simulink model "SkywalkerX8_Control_Digital"  (R2018a)
settings: Solver=FixedStepAuto  StartTime=0.0  StopTime=120  FixedStep=0.001  RelTol=1e-3
undefined symbols (not defined in the file): DiscIntNeverNeededParam, sigbuilder_block, SkywalkerX8
libraries: simulink_extras x9, simulink x3
(part 1 of 2)
settings Model: Creator=David  LastModifiedBy=David
settings OptimizationCC: DefaultParameterBehavior=Inlined  EnhancedBackFolding=on  PassReuseOutputArgsThreshold=0  OptimizeBlockOrder=speed  DifferentSizesBufferReuse=on  OptimizationCustomize=off
settings DebuggingCC: ParameterTunabilityLossMsg=error
settings SFSimCC: MATLABDynamicMemAlloc=off
settings RTWCC: GenCodeOnly=on  Description=Generic Real-Time Target  GenerateReport=on  LaunchReport=on
settings CodeAppCC: ForceParamTrailComments=on  OperatorAnnotations=on

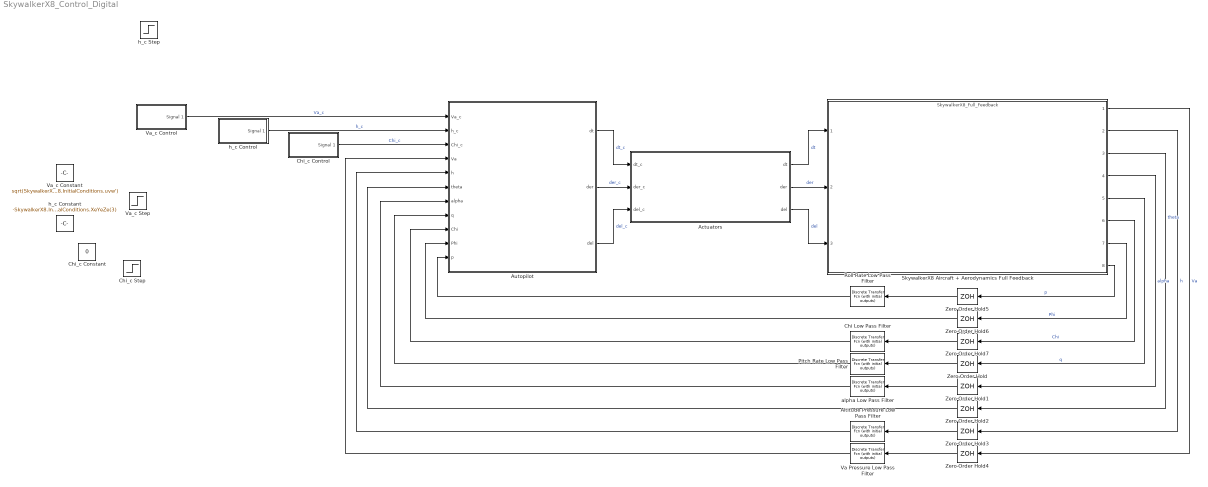
== system SkywalkerX8_Control_Digital ==
  Actuators : Subsystem
      mask Display:
      | image('actuators.jpg', 'center')
      | 
      | color('white')
      | 
      | port_label('input', 1, 'd_{t_c} (Unitless)', 'texmode', 'on')
      | port_label('input', 2, 'd_{{er}_c} (rad)', 'texmode', 'on')
      | port_label('input', 3, 'd_{{el}_c} (rad)', 'texmode', 'on')
      | 
      | port_label('output', 1, 'd_t (Unitless)', 'texmode', 'on')
      | port_label('output', 2, 'd_{er} (rad)', 'texmode', 'on')
      | port_label('output', 3, 'd_{el} (rad)', 'texmode', 'on')
  Altitude Pressure Low Pass Filter : simulink_extras/Additional Discrete/Discrete Transfer Fcn (with initial outputs)  N=cell2mat(SkywalkerX8.Sensors.Filters.AltitudePressure.FilterTFDigital.Numerator)  D=cell2mat(SkywalkerX8.Sensors.Filters.AltitudePressure.FilterTFDigital.Denominator)  U0=-SkywalkerX8.InitialConditions.XeYeZe(3)  Y0=-SkywalkerX8.InitialConditions.XeYeZe(3)  TS=SkywalkerX8.Sensors.Filters.AltitudePressure.FilterSampleTime
      settings: SourceProductName=Simulink  SourceProductBaseCode=SL
  Autopilot : Subsystem
      mask Display:
      | image('autopilot.png', 'center')
      | 
      | port_label('output', 1, '\delta_t (Unitless)', 'texmode', 'on')
      | port_label('output', 2, '\delta_e_r (rad)', 'texmode', 'on')
      | port_label('output', 3, '\delta_e_l (rad)', 'texmode', 'on')
      | 
      | port_label('input', 1, 'V_{a_c} (m/s)', 'texmode', 'on')
      | port_label('input', 2, 'h_c (m)', 'texmode', 'on')
      | port_label('input', 3, '\chi_c (rad)', 'texmode', 'on')
      | port_label('input', 4, 'V_a (m/s)', 'texmode', 'on')
      | port_label('input', 5, 'Altitude (m)', 'texmode', 'on')
      | port_label('input', 6, '\theta (rad)', 'texmode', 'on')
      | port_label('input', 7, '\alpha (rad)', 'texmode', 'on')
      | port_label('input', 8, 'q (rad/s)', 'texmode', 'on')
      | port_label('input', 9, '\chi (rad)', 'texmode', 'on')
      | port_label('input', 10, '\phi (rad)', 'texmode', 'on')
      | port_label('input', 11, 'p (rad/s)', 'texmode', 'on')
  Chi Low Pass Filter : simulink_extras/Additional Discrete/Discrete Transfer Fcn (with initial outputs)  N=cell2mat(SkywalkerX8.Sensors.EKF.GPSSmoothing.Filters.ChiFilter.TFDigital.Numerator)  D=cell2mat(SkywalkerX8.Sensors.EKF.GPSSmoothing.Filters.ChiFilter.TFDigital.Denominator)  U0=SkywalkerX8.Sensors.EKF.GPSSmoothing.Filters.ChiFilter.InitialCondition  Y0=SkywalkerX8.Sensors.EKF.GPSSmoothing.Filters.ChiFilter.InitialCondition  TS=SkywalkerX8.Sensors.EKF.GPSSmoothing.Filters.ChiFilter.SampleTime
      settings: SourceProductName=Simulink  SourceProductBaseCode=SL
  Chi_c Constant : Constant  Value=0
  Chi_c Control : Subsystem  Tag=STV Subsys  LoadFcn=sigbuilder_block('load');  StartFcn=sigbuilder_block('start');  StopFcn=sigbuilder_block('stop');  ClipboardFcn=sigbuilder_block('clipboard');  mask(Sigbuilder block){tuvar=[0:10]}
      mask help: Simulink:masks:SigbuilderBlock_MD
      mask init:
      | if ~strcmp(get_param(bdroot(gcbh),'SimulationStatus'),'stopped') tuvar = sigbuilder_block('maskInit'); end
      settings: CopyFcn=sigbuilder_block('copy');  DeleteFcn=sigbuilder_block('delete');  ModelCloseFcn=sigbuilder_block('modelClose');  PreSaveFcn=sigbuilder_block('preSave');  PauseFcn=sigbuilder_block('pause');  ContinueFcn=sigbuilder_block('continue');  NameChangeFcn=sigbuilder_block('namechange');  OpenFcn=sigbuilder_block('open',[437.6 199.2 550.4 400 ]);  CloseFcn=sigbuilder_block('close');
      mask Display: plot(0, 0, 100, 100,[2, 2, 32, 32, 2], [68, 8, 8, 68, 68],[32, 2], [38, 38], [32, 19, 2],[53, 60, 44], [32, 17, 17, 2],[16, 16, 31, 31]);txt = getActiveGroup(gcbh);text(2, 100, txt,'verticalAlignment', 'top');
  Chi_c Step : Step  After=deg2rad(90)  SampleTime=0
  Pitch Rate Low Pass Filter : simulink_extras/Additional Discrete/Discrete Transfer Fcn (with initial outputs)  N=cell2mat(SkywalkerX8.Sensors.Filters.AngularRates.Pitch.FilterTFDigital.Numerator)  D=cell2mat(SkywalkerX8.Sensors.Filters.AngularRates.Pitch.FilterTFDigital.Denominator)  U0=SkywalkerX8.Sensors.Filters.AngularRates.Pitch.InitialCondition  Y0=SkywalkerX8.Sensors.Filters.AngularRates.Pitch.InitialCondition  TS=SkywalkerX8.Sensors.Filters.AngularRates.Pitch.FilterSampleTime
      settings: SourceProductName=Simulink  SourceProductBaseCode=SL
  Roll Rate Low Pass Filter : simulink_extras/Additional Discrete/Discrete Transfer Fcn (with initial outputs)  N=cell2mat(SkywalkerX8.Sensors.Filters.AngularRates.Roll.FilterTFDigital.Numerator)  D=cell2mat(SkywalkerX8.Sensors.Filters.AngularRates.Roll.FilterTFDigital.Denominator)  U0=SkywalkerX8.Sensors.Filters.AngularRates.Roll.InitialCondition  Y0=SkywalkerX8.Sensors.Filters.AngularRates.Roll.InitialCondition  TS=SkywalkerX8.Sensors.Filters.AngularRates.Roll.FilterSampleTime
      settings: SourceProductName=Simulink  SourceProductBaseCode=SL
  SkywalkerX8 Aircraft + Aerodynamics Full Feedback : ModelReference  ModelNameDialog=SkywalkerX8_Full_Feedback  ModelReferenceVersion=1.30
      mask Display:
      | image('x8SkySunset.png', 'center')
      | 
      | port_label('input', 1, '\delta_t (Unitless)', 'texmode', 'on')
      | port_label('input', 2, '\delta_e_r (rad)', 'texmode', 'on')
      | port_label('input', 3, '\delta_e_l (rad)', 'texmode', 'on')
      | 
      | port_label('output', 1, 'V_a (m/s)', 'texmode', 'on')
      | port_label('output', 2, 'Altitude (m)', 'texmode', 'on')
      | port_label('output', 3, '\theta (rad)', 'texmode', 'on')
      | port_label('output', 4, '\alpha (rad)', 'texmode', 'on')
      | port_label('output', 5, 'q (rad/s)', 'texmode', 'on')
      | port_label('output', 6, '\chi (rad)', 'texmode', 'on')
      | port_label('output', 7, '\phi (rad)', 'texmode', 'on')
      | port_label('output', 8, 'p (rad/s)', 'texmode', 'on')
  Va Pressure Low Pass Filter : simulink_extras/Additional Discrete/Discrete Transfer Fcn (with initial outputs)  N=cell2mat(SkywalkerX8.Sensors.Filters.AirspeedPressure.FilterTFDigital.Numerator)  D=cell2mat(SkywalkerX8.Sensors.Filters.AirspeedPressure.FilterTFDigital.Denominator)  U0=sqrt(SkywalkerX8.InitialConditions.uvw*SkywalkerX8.InitialConditions.uvw')  Y0=sqrt(SkywalkerX8.InitialConditions.uvw*SkywalkerX8.InitialConditions.uvw')  TS=SkywalkerX8.Sensors.Filters.AirspeedPressure.FilterSampleTime
      settings: SourceProductName=Simulink  SourceProductBaseCode=SL
  Va_c Constant : Constant  Value=sqrt(SkywalkerX8.InitialConditions.uvw*SkywalkerX8.InitialConditions.uvw')
  Va_c Control : Subsystem  Tag=STV Subsys  LoadFcn=sigbuilder_block('load');  StartFcn=sigbuilder_block('start');  StopFcn=sigbuilder_block('stop');  ClipboardFcn=sigbuilder_block('clipboard');  mask(Sigbuilder block){tuvar=[0:10]}
      mask help: Simulink:masks:SigbuilderBlock_MD
      mask init:
      | if ~strcmp(get_param(bdroot(gcbh),'SimulationStatus'),'stopped') tuvar = sigbuilder_block('maskInit'); end
      settings: CopyFcn=sigbuilder_block('copy');  DeleteFcn=sigbuilder_block('delete');  ModelCloseFcn=sigbuilder_block('modelClose');  PreSaveFcn=sigbuilder_block('preSave');  PauseFcn=sigbuilder_block('pause');  ContinueFcn=sigbuilder_block('continue');  NameChangeFcn=sigbuilder_block('namechange');  OpenFcn=sigbuilder_block('open',[437.6 199.2 550.4 400 ]);  CloseFcn=sigbuilder_block('close');
      mask Display: plot(0, 0, 100, 100,[2, 2, 32, 32, 2], [68, 8, 8, 68, 68],[32, 2], [38, 38], [32, 19, 2],[53, 60, 44], [32, 17, 17, 2],[16, 16, 31, 31]);txt = getActiveGroup(gcbh);text(2, 100, txt,'verticalAlignment', 'top');
  Va_c Step : Step  Before=sqrt(SkywalkerX8.InitialConditions.uvw*SkywalkerX8.InitialConditions.uvw')  After=sqrt(SkywalkerX8.InitialConditions.uvw*SkywalkerX8.InitialConditions.uvw')  SampleTime=0
  Zero-Order Hold : ZeroOrderHold  SampleTime=SkywalkerX8.Sensors.IMU.Gyroscope.SampleTime
  Zero-Order Hold1 : ZeroOrderHold  SampleTime=SkywalkerX8.Sensors.AoA.SampleTime
  Zero-Order Hold2 : ZeroOrderHold  SampleTime=SkywalkerX8.Sensors.EKF.GPSSmoothing.StateTransitionSampleTime
  Zero-Order Hold3 : ZeroOrderHold  SampleTime=SkywalkerX8.Sensors.AltitudePressure.SampleTime
  Zero-Order Hold4 : ZeroOrderHold  SampleTime=SkywalkerX8.Sensors.AirspeedPressure.SampleTime
  Zero-Order Hold5 : ZeroOrderHold  SampleTime=SkywalkerX8.Sensors.IMU.Gyroscope.SampleTime
  Zero-Order Hold6 : ZeroOrderHold  SampleTime=SkywalkerX8.Sensors.EKF.Attitude.StateTransitionSampleTime
  Zero-Order Hold7 : ZeroOrderHold  SampleTime=SkywalkerX8.Sensors.EKF.GPSSmoothing.StateTransitionSampleTime
  alpha Low Pass Filter : simulink_extras/Additional Discrete/Discrete Transfer Fcn (with initial outputs)  N=cell2mat(SkywalkerX8.Sensors.Filters.AoA.FilterTFDigital.Numerator)  D=cell2mat(SkywalkerX8.Sensors.Filters.AoA.FilterTFDigital.Denominator)  U0=SkywalkerX8.Sensors.Filters.AoA.InitialCondition  Y0=SkywalkerX8.Sensors.Filters.AoA.InitialCondition  TS=SkywalkerX8.Sensors.Filters.AoA.FilterSampleTime
      settings: SourceProductName=Simulink  SourceProductBaseCode=SL
  h_c Constant : Constant  Value=-SkywalkerX8.InitialConditions.XeYeZe(3)
  h_c Control : Subsystem  Tag=STV Subsys  LoadFcn=sigbuilder_block('load');  StartFcn=sigbuilder_block('start');  StopFcn=sigbuilder_block('stop');  ClipboardFcn=sigbuilder_block('clipboard');  mask(Sigbuilder block){tuvar=[0:10]}
      mask help: Simulink:masks:SigbuilderBlock_MD
      mask init:
      | if ~strcmp(get_param(bdroot(gcbh),'SimulationStatus'),'stopped') tuvar = sigbuilder_block('maskInit'); end
      settings: CopyFcn=sigbuilder_block('copy');  DeleteFcn=sigbuilder_block('delete');  ModelCloseFcn=sigbuilder_block('modelClose');  PreSaveFcn=sigbuilder_block('preSave');  PauseFcn=sigbuilder_block('pause');  ContinueFcn=sigbuilder_block('continue');  NameChangeFcn=sigbuilder_block('namechange');  OpenFcn=sigbuilder_block('open',[6 30 1428 771.75 ]);  CloseFcn=sigbuilder_block('close');
      mask Display: plot(0, 0, 100, 100,[2, 2, 32, 32, 2], [68, 8, 8, 68, 68],[32, 2], [38, 38], [32, 19, 2],[53, 60, 44], [32, 17, 17, 2],[16, 16, 31, 31]);txt = getActiveGroup(gcbh);text(2, 100, txt,'verticalAlignment', 'top');
  h_c Step : Step  Time=0.1  Before=-SkywalkerX8.InitialConditions.XeYeZe(3)  After=100  SampleTime=0
  wires:
  SkywalkerX8 Aircraft + Aerodynamics Full Feedback/6 -> Zero-Order Hold7/1  "Chi"
  SkywalkerX8 Aircraft + Aerodynamics Full Feedback/5 -> Zero-Order Hold/1  "q"
  SkywalkerX8 Aircraft + Aerodynamics Full Feedback/4 -> Zero-Order Hold1/1  "alpha"
  SkywalkerX8 Aircraft + Aerodynamics Full Feedback/3 -> Zero-Order Hold2/1  "theta"
  SkywalkerX8 Aircraft + Aerodynamics Full Feedback/2 -> Zero-Order Hold3/1  "h"
  SkywalkerX8 Aircraft + Aerodynamics Full Feedback/1 -> Zero-Order Hold4/1  "Va"
  Zero-Order Hold5/1 -> Roll Rate Low Pass Filter/1
  Zero-Order Hold6/1 -> Autopilot/10(Phi)
  Zero-Order Hold7/1 -> Chi Low Pass Filter/1
  Zero-Order Hold/1 -> Pitch Rate Low Pass Filter/1
  Zero-Order Hold1/1 -> alpha Low Pass Filter/1
  Zero-Order Hold2/1 -> Autopilot/6(theta)
  Zero-Order Hold3/1 -> Altitude Pressure Low Pass Filter/1
  Zero-Order Hold4/1 -> Va Pressure Low Pass Filter/1
  h_c Control/1(Signal 1) -> Autopilot/2(h_c)  "h_c"
  Chi_c Control/1(Signal 1) -> Autopilot/3(Chi_c)  "Chi_c"
  Va_c Control/1(Signal 1) -> Autopilot/1(Va_c)  "Va_c"
  SkywalkerX8 Aircraft + Aerodynamics Full Feedback/8 -> Zero-Order Hold5/1  "p"
  SkywalkerX8 Aircraft + Aerodynamics Full Feedback/7 -> Zero-Order Hold6/1  "Phi"
  Autopilot/1(dt) -> Actuators/1(dt_c)  "dt_c"
  Actuators/1(dt) -> SkywalkerX8 Aircraft + Aerodynamics Full Feedback/1  "dt"
  Autopilot/2(der) -> Actuators/2(der_c)  "der_c"
  Actuators/2(der) -> SkywalkerX8 Aircraft + Aerodynamics Full Feedback/2  "der"
  Autopilot/3(del) -> Actuators/3(del_c)  "del_c"
  Actuators/3(del) -> SkywalkerX8 Aircraft + Aerodynamics Full Feedback/3  "del"
  Roll Rate Low Pass Filter/1 -> Autopilot/11(p)
  alpha Low Pass Filter/1 -> Autopilot/7(alpha)
  Altitude Pressure Low Pass Filter/1 -> Autopilot/5(h)
  Va Pressure Low Pass Filter/1 -> Autopilot/4(Va)
  Pitch Rate Low Pass Filter/1 -> Autopilot/8(q)
  Chi Low Pass Filter/1 -> Autopilot/9(Chi)

== system SkywalkerX8_Control_Digital/Actuators ==
  dt_c : Inport
  der_c : Inport  Port=2
  del_c : Inport  Port=3
  Left Servo-Motor : Subsystem
      mask Display: image('servo.jpg', 'center')
  Motor Model : simulink_extras/Additional Linear/State-Space (with initial outputs)  A=SkywalkerX8.Actuators.Motor.SS.A  B=SkywalkerX8.Actuators.Motor.SS.B  C=SkywalkerX8.Actuators.Motor.SS.C  D=SkywalkerX8.Actuators.Motor.SS.D  U0=SkywalkerX8.InitialConditions.dt  Y0=SkywalkerX8.InitialConditions.dt  mask(State-Space with Initial Outputs){}
      settings: SourceProductName=Simulink  SourceProductBaseCode=SL
      mask Display: image('motor.jpg', 'center')
  Right Servo-Motor : Subsystem
      mask Display: image('servo.jpg', 'center')
  dt : Outport
  der : Outport  Port=2
  del : Outport  Port=3
  wires:
  del_c/1 -> Left Servo-Motor/1(del_c)
  Motor Model/1 -> dt/1
  Left Servo-Motor/1(del) -> del/1
  der_c/1 -> Right Servo-Motor/1(der_c)
  dt_c/1 -> Motor Model/1
  Right Servo-Motor/1(der) -> der/1

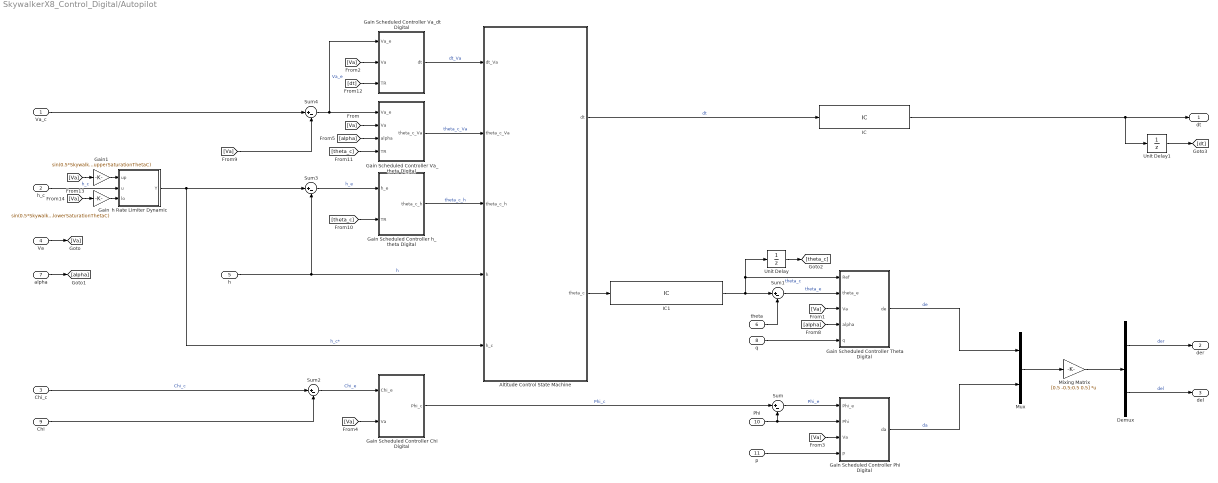
== system SkywalkerX8_Control_Digital/Autopilot ==
  Va_c : Inport
  h_c : Inport  Port=2
  Chi_c : Inport  Port=3
  Va : Inport  Port=4
  h : Inport  Port=5
  theta : Inport  Port=6
  alpha : Inport  Port=7
  q : Inport  Port=8
  Chi : Inport  Port=9
  Phi : Inport  Port=10
  p : Inport  Port=11
  Altitude Control State Machine : Stateflow chart  TreatAsAtomicUnit=on  mask{h_hold=SkywalkerX8.Control.Longitudinal.AltStateMachine.hHold, h_takeoff=SkywalkerX8.Control.Longitudinal.AltStateMachine.hTakeOff, theta_c_takeoff=SkywalkerX8.Control.Longitudinal.AltStateMachine.thetaTakeOff, hyst_frac=SkywalkerX8.Control.Longitudinal.AltStateMachine.HysteresisFraction, PreFlightBypass=SkywalkerX8.Control.Longitudinal.AltStateMachine.PreFlightBypass}
      mask prompts: h_hold "Altitude hold zone (+- band around the commanded altitude where theta will control altitude) (m)"; h_takeoff "Takeoff altitude (altitude after which we move away from constant pitch angle command) (m)"; theta_c_takeoff "Takeoff pitch angle (constant pitch angle at which to climb at at takeoff) (rad)"; hyst_frac "Hysteresis Fraction (Unitless)"; PreFlightBypass "Preflight Bypass (Unitless)"
  Demux : Demux  Outputs=2
  Gain : Gain  Gain=sin(0.5*SkywalkerX8.Control.Longitudinal.altController.lowerSaturationThetaC)
  Gain Scheduled Controller Chi Digital : Subsystem
  Gain Scheduled Controller Phi Digital : Subsystem
  Gain Scheduled Controller Theta Digital : Subsystem
  Gain Scheduled Controller Va_dt Digital : Subsystem
  Gain Scheduled Controller Va_theta Digital : Subsystem
  Gain Scheduled Controller h_theta Digital : Subsystem
  Gain1 : Gain  Gain=sin(0.5*SkywalkerX8.Control.Longitudinal.altController.upperSaturationThetaC)
  IC : InitialCondition  Value=SkywalkerX8.InitialConditions.dt
  IC1 : InitialCondition  Value=SkywalkerX8.InitialConditions.PhiThetaPsi(2)
  Mixing Matrix : Gain  Gain=[0.5 -0.5;0.5 0.5]  Multiplication=Matrix(K*u)
  Mux : Mux  Inputs=2
  Sum{,1..4} (5 alike) : Sum  Inputs=|+-
  Unit Delay : UnitDelay  InitialCondition=SkywalkerX8.InitialConditions.PhiThetaPsi(2)  SampleTime=SkywalkerX8.Control.Longitudinal.thetaController.Digital.SampleTime
  Unit Delay1 : UnitDelay  InitialCondition=SkywalkerX8.InitialConditions.dt  SampleTime=SkywalkerX8.Control.Longitudinal.VaDtController.Digital.SampleTime
  h Rate Limiter Dynamic : Subsystem  mask{initOutput=-SkywalkerX8.InitialConditions.XeYeZe(3)}
      mask prompts: initOutput "Initial output of dynamic rate limiter"
      mask DialogControl DescGroupVar Prompt: Rate Limiter Dynamic
      mask DialogControl DescTextVar Prompt: Limit rising and falling rates of the signals at the second input by using the first input (upper limit) and the third input (lower limit).
      mask Display:
      | image('rateLimit.png')
      | 
      | port_label('input', 1, 'up')
      | port_label('input', 2, 'u')
      | port_label('input', 3, 'lo')
      | 
      | port_label('output', 1, 'Y')
  dt : Outport
  der : Outport  Port=2
  del : Outport  Port=3
  wires:
  [Va] -> Sum4/2
  Sum4/1 -> Gain Scheduled Controller Va_theta Digital/1(Va_e), Gain Scheduled Controller Va_dt Digital/1(Va_e)  "Va_e"
  Demux/1 -> der/1  "der"
  Gain Scheduled Controller Chi Digital/1(Phi_c) -> Sum/1  "Phi_c"
  h/1 -> Altitude Control State Machine/4(h), Sum3/2  "h"
  h Rate Limiter Dynamic/1(Y) -> Altitude Control State Machine/5(h_c), Sum3/1  "h_c*"
  Sum3/1 -> Gain Scheduled Controller h_theta Digital/1(h_e)  "h_e"
  Sum2/1 -> Gain Scheduled Controller Chi Digital/1(Chi_e)  "Chi_e"
  Phi/1 -> Gain Scheduled Controller Phi Digital/2(Phi), Sum/2
  Sum/1 -> Gain Scheduled Controller Phi Digital/1(Phi_e)  "Phi_e"
  Gain Scheduled Controller Phi Digital/1(da) -> Mux/2  "da"
  [Va] -> Gain Scheduled Controller Phi Digital/3(Va)
  [Va] -> Gain Scheduled Controller Theta Digital/3(Va)
  [alpha] -> Gain Scheduled Controller Va_theta Digital/3(alpha)
  [Va] -> Gain Scheduled Controller Chi Digital/2(Va)
  Sum1/1 -> Gain Scheduled Controller Theta Digital/2(theta_e)  "theta_e"
  [Va] -> Gain Scheduled Controller Va_dt Digital/2(Va)
  Demux/2 -> del/1  "del"
  alpha/1 -> [alpha]
  [Va] -> Gain Scheduled Controller Va_theta Digital/2(Va)
  Chi/1 -> Sum2/2
  Gain Scheduled Controller Theta Digital/1(de) -> Mux/1  "de"
  p/1 -> Gain Scheduled Controller Phi Digital/4(p)
  Va/1 -> [Va]
  theta/1 -> Sum1/2
  Mux/1 -> Mixing Matrix/1
  Mixing Matrix/1 -> Demux/1
  Altitude Control State Machine/1(dt) -> IC/1  "dt"
  Gain Scheduled Controller Va_theta Digital/1(theta_c_Va) -> Altitude Control State Machine/2(theta_c_Va)  "theta_c_Va"
  [theta_c] -> Gain Scheduled Controller Va_theta Digital/4(TR)
  [dt] -> Gain Scheduled Controller Va_dt Digital/3(TR)
  IC/1 -> Unit Delay1/1, dt/1
  [theta_c] -> Gain Scheduled Controller h_theta Digital/2(TR)
  IC1/1 -> Gain Scheduled Controller Theta Digital/1(Ref), Unit Delay/1, Sum1/1  "theta_c"
  [alpha] -> Gain Scheduled Controller Theta Digital/4(alpha)
  q/1 -> Gain Scheduled Controller Theta Digital/5(q)
  Gain Scheduled Controller h_theta Digital/1(theta_c_h) -> Altitude Control State Machine/3(theta_c_h)  "theta_c_h"
  Altitude Control State Machine/2(theta_c) -> IC1/1
  Gain Scheduled Controller Va_dt Digital/1(dt) -> Altitude Control State Machine/1(dt_Va)  "dt_Va"
  h_c/1 -> h Rate Limiter Dynamic/2(u)  "h_c"
  [Va] -> Gain1/1
  Gain/1 -> h Rate Limiter Dynamic/3(lo)
  [Va] -> Gain/1
  Gain1/1 -> h Rate Limiter Dynamic/1(up)
  Chi_c/1 -> Sum2/1  "Chi_c"
  Va_c/1 -> Sum4/1
  Unit Delay/1 -> [theta_c]
  Unit Delay1/1 -> [dt]

== system SkywalkerX8_Control_Digital/Chi_c Control ==
  Demux : Demux  Tag=STV Demux  Outputs=1
  FromWs : FromWorkspace  Tag=STV FromWs  VariableName=tuvar  SampleTime=0
      SigBuilderData=|
      | common.afterFinalStr = 'Extrapolate'
      | common.sampleTime = 0
      | dataSet.timeRange = [0 120]
      | dataSet.name = 'Group 1'
      | sbobj.Groups.Name = 'Group 1'
      | sbobj.Groups.Signals.Name = 'Signal 1'
      | sbobj.Groups.Signals.XData = [0 10 10 35 35 55 55 90 90 120]
      | sbobj.Groups.Signals.YData = [0 0 1.5708 1.5708 0 0 1.5708 1.5708 0 0]
      | sbobj.Groups.TimeRange = [0 120]
  Signal 1 : Outport  Tag=STV Outport
  wires:
  Demux/1 -> Signal 1/1
  FromWs/1 -> Demux/1

== system SkywalkerX8_Control_Digital/Va_c Control ==
  Demux : Demux  Tag=STV Demux  Outputs=1
  FromWs : FromWorkspace  Tag=STV FromWs  VariableName=tuvar  SampleTime=0
      SigBuilderData=|
      | common.afterFinalStr = 'Extrapolate'
      | common.sampleTime = 0
      | dataSet.timeRange = [0 120]
      | dataSet.name = 'Group 1'
      | sbobj.Groups.Name = 'Group 1'
      | sbobj.Groups.Signals.Name = 'Signal 1'
      | sbobj.Groups.Signals.XData = [0 10 10 30 30 50 50 70 70 120]
      | sbobj.Groups.Signals.YData = [17.3072 17.3 20 20 17.3072 17.3072 15 15 17.3072 17.3072]
      | sbobj.Groups.TimeRange = [0 120]
  Signal 1 : Outport  Tag=STV Outport
  wires:
  Demux/1 -> Signal 1/1
  FromWs/1 -> Demux/1

== system SkywalkerX8_Control_Digital/h_c Control ==
  Demux : Demux  Tag=STV Demux  Outputs=1
  FromWs : FromWorkspace  Tag=STV FromWs  VariableName=tuvar  SampleTime=0
      SigBuilderData=|
      | common.afterFinalStr = 'Extrapolate'
      | common.sampleTime = 0
      | dataSet.timeRange = [0 120]
      | dataSet.name = 'Group 1'
      | sbobj.Groups.Name = 'Group 1'
      | sbobj.Groups.Signals.Name = 'Signal 1'
      | sbobj.Groups.Signals.XData = [0 1 1 20 20 40 40 60 80 80 100 100 120]
      | sbobj.Groups.Signals.YData = [50 50 60 60 75 75 100 100 80 60 60 100 100]
      | sbobj.Groups.TimeRange = [0 120]
  Signal 1 : Outport  Tag=STV Outport
  wires:
  Demux/1 -> Signal 1/1
  FromWs/1 -> Demux/1

== system SkywalkerX8_Control_Digital/Actuators/Left Servo-Motor ==
  del_c : Inport
  Abs : Abs
  Compare To Constant : simulink/Logic and Bit Operations/Compare To Constant  relop=>  const=SkywalkerX8.Actuators.Servos.RateLimit  OutDataTypeStr=boolean
  Derivative : Derivative
  Rate Limiter : RateLimiter  Commented=through  RisingSlewLimit=SkywalkerX8.Actuators.Servos.RateLimit  FallingSlewLimit=-SkywalkerX8.Actuators.Servos.RateLimit  SampleTimeMode=inherited  InitialCondition=SkywalkerX8.InitialConditions.de*0.5 + SkywalkerX8.InitialConditions.da*0.5
  Saturation : Saturate  UpperLimit=SkywalkerX8.Actuators.Servos.UpperSaturation  LowerLimit=SkywalkerX8.Actuators.Servos.LowerSaturation
  Second Order Servo-Motor Model : simulink_extras/Additional Linear/State-Space (with initial outputs)  A=SkywalkerX8.Actuators.Servos.SS.A  B=SkywalkerX8.Actuators.Servos.SS.B  C=SkywalkerX8.Actuators.Servos.SS.C  D=SkywalkerX8.Actuators.Servos.SS.D  U0=(SkywalkerX8.InitialConditions.de*0.5 + SkywalkerX8.InitialConditions.da*0.5)  Y0=(SkywalkerX8.InitialConditions.de*0.5 + SkywalkerX8.InitialConditions.da*0.5)
      settings: SourceProductName=Simulink  SourceProductBaseCode=SL
  Terminator : Terminator
  del : Outport
  wires:
  Rate Limiter/1 -> Saturation/1
  del_c/1 -> Second Order Servo-Motor Model/1
  Saturation/1 -> del/1
  Derivative/1 -> Abs/1
  Abs/1 -> Compare To Constant/1
  Compare To Constant/1 -> Terminator/1  "lServoRateLimitCheck"
  Second Order Servo-Motor Model/1 -> Derivative/1, Rate Limiter/1

== system SkywalkerX8_Control_Digital/Actuators/Right Servo-Motor ==
  der_c : Inport
  Abs : Abs
  Compare To Constant : simulink/Logic and Bit Operations/Compare To Constant  relop=>  const=SkywalkerX8.Actuators.Servos.RateLimit  OutDataTypeStr=boolean
  Derivative : Derivative
  Rate Limiter : RateLimiter  Commented=through  RisingSlewLimit=SkywalkerX8.Actuators.Servos.RateLimit  FallingSlewLimit=-SkywalkerX8.Actuators.Servos.RateLimit  SampleTimeMode=inherited  InitialCondition=SkywalkerX8.InitialConditions.de*0.5 - SkywalkerX8.InitialConditions.da*0.5
  Saturation : Saturate  UpperLimit=SkywalkerX8.Actuators.Servos.UpperSaturation  LowerLimit=SkywalkerX8.Actuators.Servos.LowerSaturation
  Second Order Servo-Motor Model : simulink_extras/Additional Linear/State-Space (with initial outputs)  A=SkywalkerX8.Actuators.Servos.SS.A  B=SkywalkerX8.Actuators.Servos.SS.B  C=SkywalkerX8.Actuators.Servos.SS.C  D=SkywalkerX8.Actuators.Servos.SS.D  U0=(SkywalkerX8.InitialConditions.de*0.5 - SkywalkerX8.InitialConditions.da*0.5)  Y0=(SkywalkerX8.InitialConditions.de*0.5 - SkywalkerX8.InitialConditions.da*0.5)
      settings: SourceProductName=Simulink  SourceProductBaseCode=SL
  Terminator : Terminator
  der : Outport
  wires:
  Rate Limiter/1 -> Saturation/1
  der_c/1 -> Second Order Servo-Motor Model/1
  Second Order Servo-Motor Model/1 -> Derivative/1, Rate Limiter/1
  Saturation/1 -> der/1
  Derivative/1 -> Abs/1
  Abs/1 -> Compare To Constant/1
  Compare To Constant/1 -> Terminator/1  "rServoRateLimitCheck"

== system SkywalkerX8_Control_Digital/Autopilot/Gain Scheduled Controller Chi Digital ==
  Chi_e : Inport
  Va : Inport  Port=2
  PIDF Controller Chi Ki 2D Lookup Table : Lookup_n-D  NumberOfTableDimensions=1  BreakpointsForDimension1=SkywalkerX8.Control.Lateral.SchedulingVariables.VaArray  BreakpointsForDimension2=SkywalkerX8.Control.Longitudinal.SchedulingVariables.alphaArray  Table=SkywalkerX8.Control.Lateral.ChiController.Digital.KiChi  InternalRulePriority=Speed  RndMeth=Simplest  InputSameDT=on
  PIDF Controller Chi Kp 2D Lookup Table : Lookup_n-D  NumberOfTableDimensions=1  BreakpointsForDimension1=SkywalkerX8.Control.Lateral.SchedulingVariables.VaArray  BreakpointsForDimension2=SkywalkerX8.Control.Longitudinal.SchedulingVariables.alphaArray  Table=SkywalkerX8.Control.Lateral.ChiController.Digital.KpChi  InternalRulePriority=Speed  RndMeth=Simplest  InputSameDT=on
  PIDF Controller Va_theta : Subsystem
  Saturation : Saturate  UpperLimit=SkywalkerX8.Control.Lateral.ChiController.upperSaturationPhiC  LowerLimit=SkywalkerX8.Control.Lateral.ChiController.lowerSaturationPhiC
  Zero-Order Hold : ZeroOrderHold  SampleTime=SkywalkerX8.Control.Lateral.ChiController.Digital.SampleTime
  Phi_c : Outport
  wires:
  PIDF Controller Chi Kp 2D Lookup Table/1 -> PIDF Controller Va_theta/2(P)
  Chi_e/1 -> PIDF Controller Va_theta/1(u)
  Va/1 -> PIDF Controller Chi Kp 2D Lookup Table/1, PIDF Controller Chi Ki 2D Lookup Table/1
  PIDF Controller Chi Ki 2D Lookup Table/1 -> PIDF Controller Va_theta/3(I)
  Saturation/1 -> PIDF Controller Va_theta/4(Post-Saturation), Zero-Order Hold/1
  PIDF Controller Va_theta/1(y) -> PIDF Controller Va_theta/5(Pre-Saturation), Saturation/1
  Zero-Order Hold/1 -> Phi_c/1

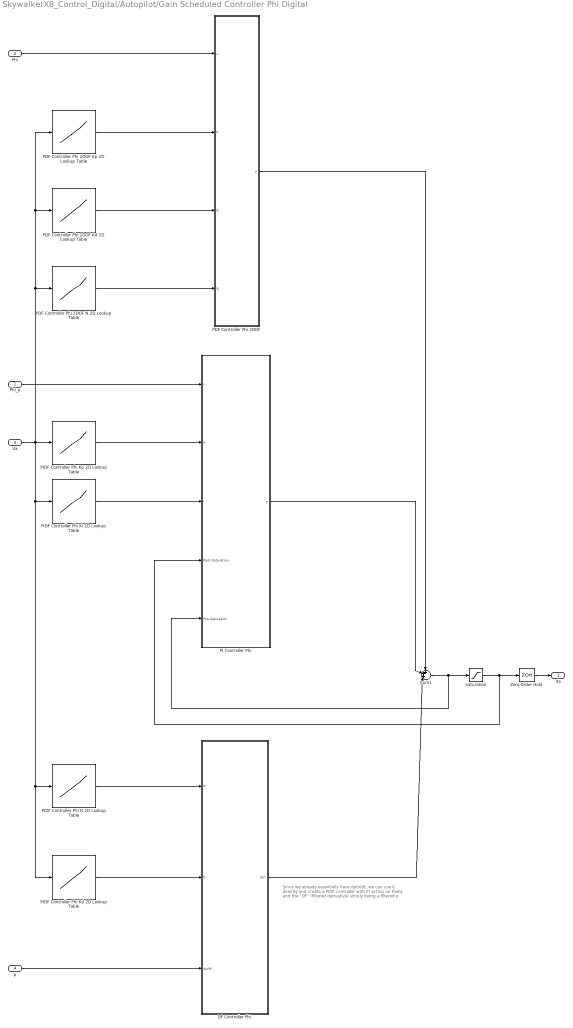
== system SkywalkerX8_Control_Digital/Autopilot/Gain Scheduled Controller Phi Digital ==
  note: Since we already essentially have dphi/dt,
      | we can use it directly and create a PIDF controller
      | with PI acting on theta and the "DF" (filtered derivative)
      | simply being a filtered p
  Phi_e : Inport
  Phi : Inport  Port=2
  Va : Inport  Port=3
  p : Inport  Port=4
  DF Controller Phi : Subsystem
  PDF Controller Phi 2DOF : Subsystem
  PDF Controller Phi 2DOF Kd 2D Lookup Table : Lookup_n-D  NumberOfTableDimensions=1  BreakpointsForDimension1=SkywalkerX8.Control.Lateral.SchedulingVariables.VaArray  BreakpointsForDimension2=SkywalkerX8.Control.Longitudinal.SchedulingVariables.alphaArray  Table=SkywalkerX8.Control.Lateral.PhiController.Digital.KdPhi2DOF  InternalRulePriority=Speed  RndMeth=Simplest  InputSameDT=on
  PDF Controller Phi 2DOF Kp 2D Lookup Table : Lookup_n-D  NumberOfTableDimensions=1  BreakpointsForDimension1=SkywalkerX8.Control.Lateral.SchedulingVariables.VaArray  BreakpointsForDimension2=SkywalkerX8.Control.Longitudinal.SchedulingVariables.alphaArray  Table=SkywalkerX8.Control.Lateral.PhiController.Digital.KpPhi2DOF  InternalRulePriority=Speed  RndMeth=Simplest  InputSameDT=on
  PDF Controller Phi 2DOF N 2D Lookup Table : Lookup_n-D  NumberOfTableDimensions=1  BreakpointsForDimension1=SkywalkerX8.Control.Lateral.SchedulingVariables.VaArray  BreakpointsForDimension2=SkywalkerX8.Control.Longitudinal.SchedulingVariables.alphaArray  Table=SkywalkerX8.Control.Lateral.PhiController.Digital.NPhi2DOF  InternalRulePriority=Speed  RndMeth=Simplest  InputSameDT=on
  PI Controller Phi : Subsystem
  PIDF Controller Phi Kd 2D Lookup Table : Lookup_n-D  NumberOfTableDimensions=1  BreakpointsForDimension1=SkywalkerX8.Control.Lateral.SchedulingVariables.VaArray  BreakpointsForDimension2=SkywalkerX8.Control.Longitudinal.SchedulingVariables.alphaArray  Table=SkywalkerX8.Control.Lateral.PhiController.Digital.KdPhi  InternalRulePriority=Speed  RndMeth=Simplest  InputSameDT=on
  PIDF Controller Phi Ki 2D Lookup Table : Lookup_n-D  NumberOfTableDimensions=1  BreakpointsForDimension1=SkywalkerX8.Control.Lateral.SchedulingVariables.VaArray  BreakpointsForDimension2=SkywalkerX8.Control.Longitudinal.SchedulingVariables.alphaArray  Table=SkywalkerX8.Control.Lateral.PhiController.Digital.KiPhi  InternalRulePriority=Speed  RndMeth=Simplest  InputSameDT=on
  PIDF Controller Phi Kp 2D Lookup Table : Lookup_n-D  NumberOfTableDimensions=1  BreakpointsForDimension1=SkywalkerX8.Control.Lateral.SchedulingVariables.VaArray  BreakpointsForDimension2=SkywalkerX8.Control.Longitudinal.SchedulingVariables.alphaArray  Table=SkywalkerX8.Control.Lateral.PhiController.Digital.KpPhi  InternalRulePriority=Speed  RndMeth=Simplest  InputSameDT=on
  PIDF Controller Phi N 2D Lookup Table : Lookup_n-D  NumberOfTableDimensions=1  BreakpointsForDimension1=SkywalkerX8.Control.Lateral.SchedulingVariables.VaArray  BreakpointsForDimension2=SkywalkerX8.Control.Longitudinal.SchedulingVariables.alphaArray  Table=SkywalkerX8.Control.Lateral.PhiController.Digital.NPhi  InternalRulePriority=Speed  RndMeth=Simplest  InputSameDT=on
  Saturation : Saturate  UpperLimit=SkywalkerX8.Control.Lateral.PhiController.upperSaturationDa  LowerLimit=SkywalkerX8.Control.Lateral.PhiController.lowerSaturationDa
  Sum1 : Sum  Inputs=+++|
  Zero-Order Hold : ZeroOrderHold  SampleTime=SkywalkerX8.Control.Lateral.PhiController.Digital.SampleTime
  da : Outport
  wires:
  Va/1 -> PDF Controller Phi 2DOF Kp 2D Lookup Table/1, PDF Controller Phi 2DOF Kd 2D Lookup Table/1, PDF Controller Phi 2DOF N 2D Lookup Table/1, PIDF Controller Phi N 2D Lookup Table/1, PIDF Controller Phi Kd 2D Lookup Table/1, PIDF Controller Phi Ki 2D Lookup Table/1, PIDF Controller Phi Kp 2D Lookup Table/1
  Phi_e/1 -> PI Controller Phi/1(u)
  PIDF Controller Phi Kp 2D Lookup Table/1 -> PI Controller Phi/2(P)
  PIDF Controller Phi Ki 2D Lookup Table/1 -> PI Controller Phi/3(I)
  PI Controller Phi/1(y) -> Sum1/2
  Sum1/1 -> Saturation/1, PI Controller Phi/5(Pre-Saturation)
  p/1 -> DF Controller Phi/3(du/dt)
  DF Controller Phi/1(da*) -> Sum1/3
  PIDF Controller Phi N 2D Lookup Table/1 -> DF Controller Phi/1(N)
  PIDF Controller Phi Kd 2D Lookup Table/1 -> DF Controller Phi/2(D)
  Saturation/1 -> Zero-Order Hold/1, PI Controller Phi/4(Post-Saturation)
  PDF Controller Phi 2DOF Kp 2D Lookup Table/1 -> PDF Controller Phi 2DOF/2(P)
  PDF Controller Phi 2DOF Kd 2D Lookup Table/1 -> PDF Controller Phi 2DOF/3(D)
  PDF Controller Phi 2DOF N 2D Lookup Table/1 -> PDF Controller Phi 2DOF/4(N)
  Phi/1 -> PDF Controller Phi 2DOF/1(u)
  PDF Controller Phi 2DOF/1(y) -> Sum1/1
  Zero-Order Hold/1 -> da/1

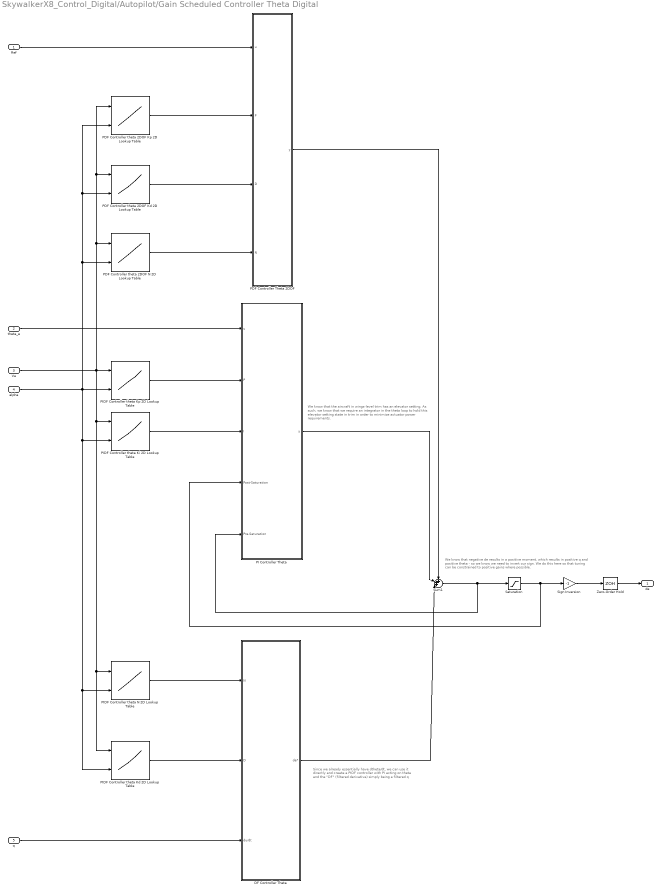
== system SkywalkerX8_Control_Digital/Autopilot/Gain Scheduled Controller Theta Digital ==
  note: Since we already essentially have dtheta/dt,
      | we can use it directly and create a PIDF controller
      | with PI acting on theta and the "DF" (filtered derivative)
      | simply being a filtered q
  note: We know that negative de results in a positive moment, which results in
      | positive q and positive theta - so we know we need to invert our sign.
      | We do this here so that tuning can be constrained to positive gains where possible.
  note: We know that the aircraft in wings-level trim has an elevator setting. As such, we know that we require an integrator in the theta loop to hold this elevator setting state in trim in order to minimize actuator power requirements.
  Ref : Inport
  theta_e : Inport  Port=2
  Va : Inport  Port=3
  alpha : Inport  Port=4
  q : Inport  Port=5
  DF Controller Theta : Subsystem
  PDF Controller Theta 2DOF : Subsystem
  PDF Controller theta 2DOF Kd 2D Lookup Table : Lookup_n-D  BreakpointsForDimension1=SkywalkerX8.Control.Longitudinal.SchedulingVariables.VaArray  BreakpointsForDimension2=SkywalkerX8.Control.Longitudinal.SchedulingVariables.alphaArray  BeginIndexSearchUsingPreviousIndexResult=on  Table=SkywalkerX8.Control.Longitudinal.thetaController.Digital.KdTheta2DOF  InternalRulePriority=Speed  RndMeth=Simplest  InputSameDT=on
  PDF Controller theta 2DOF Kp 2D Lookup Table : Lookup_n-D  BreakpointsForDimension1=SkywalkerX8.Control.Longitudinal.SchedulingVariables.VaArray  BreakpointsForDimension2=SkywalkerX8.Control.Longitudinal.SchedulingVariables.alphaArray  Table=SkywalkerX8.Control.Longitudinal.thetaController.Digital.KpTheta2DOF  InternalRulePriority=Speed  RndMeth=Simplest  InputSameDT=on
  PDF Controller theta 2DOF N 2D Lookup Table : Lookup_n-D  BreakpointsForDimension1=SkywalkerX8.Control.Longitudinal.SchedulingVariables.VaArray  BreakpointsForDimension2=SkywalkerX8.Control.Longitudinal.SchedulingVariables.alphaArray  Table=SkywalkerX8.Control.Longitudinal.thetaController.Digital.NTheta2DOF  InternalRulePriority=Speed  RndMeth=Simplest  InputSameDT=on
  PI Controller Theta : Subsystem
  PIDF Controller theta Kd 2D Lookup Table : Lookup_n-D  BreakpointsForDimension1=SkywalkerX8.Control.Longitudinal.SchedulingVariables.VaArray  BreakpointsForDimension2=SkywalkerX8.Control.Longitudinal.SchedulingVariables.alphaArray  Table=SkywalkerX8.Control.Longitudinal.thetaController.Digital.KdTheta  InternalRulePriority=Speed  RndMeth=Simplest  InputSameDT=on
  PIDF Controller theta Ki 2D Lookup Table : Lookup_n-D  BreakpointsForDimension1=SkywalkerX8.Control.Longitudinal.SchedulingVariables.VaArray  BreakpointsForDimension2=SkywalkerX8.Control.Longitudinal.SchedulingVariables.alphaArray  Table=SkywalkerX8.Control.Longitudinal.thetaController.Digital.KiTheta  InternalRulePriority=Speed  RndMeth=Simplest  InputSameDT=on
  PIDF Controller theta Kp 2D Lookup Table : Lookup_n-D  BreakpointsForDimension1=SkywalkerX8.Control.Longitudinal.SchedulingVariables.VaArray  BreakpointsForDimension2=SkywalkerX8.Control.Longitudinal.SchedulingVariables.alphaArray  Table=SkywalkerX8.Control.Longitudinal.thetaController.Digital.KpTheta  InternalRulePriority=Speed  RndMeth=Simplest  InputSameDT=on
  PIDF Controller theta N 2D Lookup Table : Lookup_n-D  BreakpointsForDimension1=SkywalkerX8.Control.Longitudinal.SchedulingVariables.VaArray  BreakpointsForDimension2=SkywalkerX8.Control.Longitudinal.SchedulingVariables.alphaArray  Table=SkywalkerX8.Control.Longitudinal.thetaController.Digital.NTheta  InternalRulePriority=Speed  RndMeth=Simplest  InputSameDT=on
  Saturation : Saturate  UpperLimit=SkywalkerX8.Control.Longitudinal.thetaController.Digital.upperSaturationNegativeDe  LowerLimit=SkywalkerX8.Control.Longitudinal.thetaController.Digital.lowerSaturationNegativeDe
  Sign Inversion : Gain  Gain=-1
  Sum1 : Sum  Inputs=+++|
  Zero-Order Hold : ZeroOrderHold  SampleTime=SkywalkerX8.Control.Longitudinal.thetaController.Digital.SampleTime
  de : Outport
  wires:
  Va/1 -> PDF Controller theta 2DOF Kd 2D Lookup Table/1, PDF Controller theta 2DOF Kp 2D Lookup Table/1, PDF Controller theta 2DOF N 2D Lookup Table/1, PIDF Controller theta N 2D Lookup Table/1, PIDF Controller theta Kd 2D Lookup Table/1, PIDF Controller theta Ki 2D Lookup Table/1, PIDF Controller theta Kp 2D Lookup Table/1
  theta_e/1 -> PI Controller Theta/1(u)
  PIDF Controller theta Kp 2D Lookup Table/1 -> PI Controller Theta/2(P)
  PIDF Controller theta Ki 2D Lookup Table/1 -> PI Controller Theta/3(I)
  alpha/1 -> PDF Controller theta 2DOF N 2D Lookup Table/2, PDF Controller theta 2DOF Kd 2D Lookup Table/2, PDF Controller theta 2DOF Kp 2D Lookup Table/2, PIDF Controller theta N 2D Lookup Table/2, PIDF Controller theta Kd 2D Lookup Table/2, PIDF Controller theta Ki 2D Lookup Table/2, PIDF Controller theta Kp 2D Lookup Table/2
  PI Controller Theta/1(y) -> Sum1/2
  Sum1/1 -> Saturation/1, PI Controller Theta/5(Pre-Saturation)
  Saturation/1 -> Sign Inversion/1, PI Controller Theta/4(Post-Saturation)
  PIDF Controller theta N 2D Lookup Table/1 -> DF Controller Theta/1(N)
  PIDF Controller theta Kd 2D Lookup Table/1 -> DF Controller Theta/2(D)
  q/1 -> DF Controller Theta/3(du/dt)
  DF Controller Theta/1(de*) -> Sum1/3
  Sign Inversion/1 -> Zero-Order Hold/1
  PDF Controller theta 2DOF Kp 2D Lookup Table/1 -> PDF Controller Theta 2DOF/2(P)
  PDF Controller theta 2DOF Kd 2D Lookup Table/1 -> PDF Controller Theta 2DOF/3(D)
  PDF Controller theta 2DOF N 2D Lookup Table/1 -> PDF Controller Theta 2DOF/4(N)
  Ref/1 -> PDF Controller Theta 2DOF/1(u)
  PDF Controller Theta 2DOF/1(y) -> Sum1/1
  Zero-Order Hold/1 -> de/1

== system SkywalkerX8_Control_Digital/Autopilot/Gain Scheduled Controller Va_dt Digital ==
  Va_e : Inport
  Va : Inport  Port=2
  TR : Inport  Port=3
  PIDF Controller Va_dt : Subsystem
  PIDF Controller Va_dt Kd Lookup Table : Lookup_n-D  NumberOfTableDimensions=1  BreakpointsForDimension1=SkywalkerX8.Control.Longitudinal.SchedulingVariables.VaArray  BreakpointsForDimension2=[1 2 3 4 5]  Table=SkywalkerX8.Control.Longitudinal.VaDtController.Digital.KdVaDt  InternalRulePriority=Speed  RndMeth=Simplest  InputSameDT=on
  PIDF Controller Va_dt Ki Lookup Table : Lookup_n-D  NumberOfTableDimensions=1  BreakpointsForDimension1=SkywalkerX8.Control.Longitudinal.SchedulingVariables.VaArray  BreakpointsForDimension2=[1 2 3 4 5]  Table=SkywalkerX8.Control.Longitudinal.VaDtController.Digital.KiVaDt  InternalRulePriority=Speed  RndMeth=Simplest  InputSameDT=on
  PIDF Controller Va_dt Kp Lookup Table : Lookup_n-D  NumberOfTableDimensions=1  BreakpointsForDimension1=SkywalkerX8.Control.Longitudinal.SchedulingVariables.VaArray  BreakpointsForDimension2=[1 2 3 4 5]  Table=SkywalkerX8.Control.Longitudinal.VaDtController.Digital.KpVaDt  InternalRulePriority=Speed  RndMeth=Simplest  InputSameDT=on
  PIDF Controller Va_dt Kt Tracking Gain Scalar : Gain  Gain=SkywalkerX8.Control.Longitudinal.VaDtController.KtScalar
  PIDF Controller Va_dt N Lookup Table : Lookup_n-D  NumberOfTableDimensions=1  BreakpointsForDimension1=SkywalkerX8.Control.Longitudinal.SchedulingVariables.VaArray  BreakpointsForDimension2=[1 2 3 4 5]  Table=SkywalkerX8.Control.Longitudinal.VaDtController.Digital.NVaDt  InternalRulePriority=Speed  RndMeth=Simplest  InputSameDT=on
  Zero-Order Hold : ZeroOrderHold  SampleTime=SkywalkerX8.Control.Longitudinal.VaDtController.Digital.SampleTime
  dt : Outport
  wires:
  Va_e/1 -> PIDF Controller Va_dt/1(u)
  PIDF Controller Va_dt/1(y) -> Zero-Order Hold/1
  PIDF Controller Va_dt Kp Lookup Table/1 -> PIDF Controller Va_dt/2(P)
  Va/1 -> PIDF Controller Va_dt Kp Lookup Table/1, PIDF Controller Va_dt Ki Lookup Table/1, PIDF Controller Va_dt N Lookup Table/1, PIDF Controller Va_dt Kd Lookup Table/1
  PIDF Controller Va_dt Ki Lookup Table/1 -> PIDF Controller Va_dt/3(I), PIDF Controller Va_dt Kt Tracking Gain Scalar/1
  PIDF Controller Va_dt Kd Lookup Table/1 -> PIDF Controller Va_dt/4(D)
  PIDF Controller Va_dt N Lookup Table/1 -> PIDF Controller Va_dt/5(N)
  TR/1 -> PIDF Controller Va_dt/7(TR)
  PIDF Controller Va_dt Kt Tracking Gain Scalar/1 -> PIDF Controller Va_dt/6(Kt)
  Zero-Order Hold/1 -> dt/1

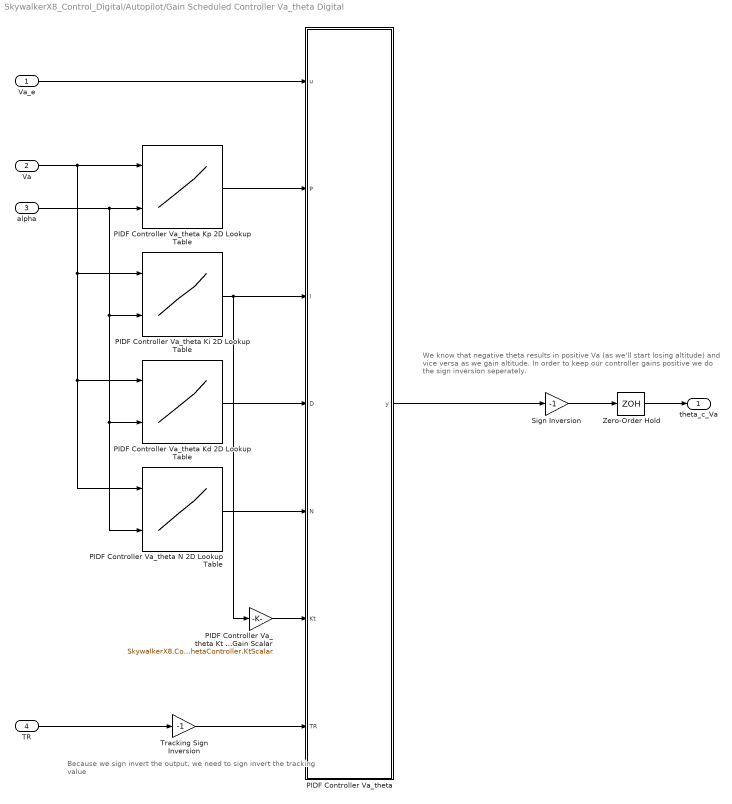
== system SkywalkerX8_Control_Digital/Autopilot/Gain Scheduled Controller Va_theta Digital ==
  note: We know that negative theta results in positive Va (as we'll start losing altitude)
      | and vice versa as we gain altitude. In order to keep our controller gains positive
      |  we do the sign inversion seperately.
  note: Because we sign invert the output, we need to sign invert the tracking
      | value
  Va_e : Inport
  Va : Inport  Port=2
  alpha : Inport  Port=3
  TR : Inport  Port=4
  PIDF Controller Va_theta : Subsystem
  PIDF Controller Va_theta Kd 2D Lookup Table : Lookup_n-D  BreakpointsForDimension1=SkywalkerX8.Control.Longitudinal.SchedulingVariables.VaArray  BreakpointsForDimension2=SkywalkerX8.Control.Longitudinal.SchedulingVariables.alphaArray  Table=SkywalkerX8.Control.Longitudinal.VaThetaController.Digital.KdVaTheta  InternalRulePriority=Speed  RndMeth=Simplest  InputSameDT=on
  PIDF Controller Va_theta Ki 2D Lookup Table : Lookup_n-D  BreakpointsForDimension1=SkywalkerX8.Control.Longitudinal.SchedulingVariables.VaArray  BreakpointsForDimension2=SkywalkerX8.Control.Longitudinal.SchedulingVariables.alphaArray  Table=SkywalkerX8.Control.Longitudinal.VaThetaController.Digital.KiVaTheta  InternalRulePriority=Speed  RndMeth=Simplest  InputSameDT=on
  PIDF Controller Va_theta Kp 2D Lookup Table : Lookup_n-D  BreakpointsForDimension1=SkywalkerX8.Control.Longitudinal.SchedulingVariables.VaArray  BreakpointsForDimension2=SkywalkerX8.Control.Longitudinal.SchedulingVariables.alphaArray  Table=SkywalkerX8.Control.Longitudinal.VaThetaController.Digital.KpVaTheta  InternalRulePriority=Speed  RndMeth=Simplest  InputSameDT=on
  PIDF Controller Va_theta Kt Tracking Gain Scalar : Gain  Gain=SkywalkerX8.Control.Longitudinal.VaThetaController.KtScalar
  PIDF Controller Va_theta N 2D Lookup Table : Lookup_n-D  BreakpointsForDimension1=SkywalkerX8.Control.Longitudinal.SchedulingVariables.VaArray  BreakpointsForDimension2=SkywalkerX8.Control.Longitudinal.SchedulingVariables.alphaArray  Table=SkywalkerX8.Control.Longitudinal.VaThetaController.Digital.NVaTheta  InternalRulePriority=Speed  RndMeth=Simplest  InputSameDT=on
  Sign Inversion : Gain  Gain=-1
  Tracking Sign Inversion : Gain  Gain=-1
  Zero-Order Hold : ZeroOrderHold  SampleTime=SkywalkerX8.Control.Longitudinal.altController.Digital.SampleTime
  theta_c_Va : Outport
  wires:
  Va_e/1 -> PIDF Controller Va_theta/1(u)
  PIDF Controller Va_theta/1(y) -> Sign Inversion/1
  PIDF Controller Va_theta Kp 2D Lookup Table/1 -> PIDF Controller Va_theta/2(P)
  Va/1 -> PIDF Controller Va_theta Kp 2D Lookup Table/1, PIDF Controller Va_theta Ki 2D Lookup Table/1, PIDF Controller Va_theta N 2D Lookup Table/1, PIDF Controller Va_theta Kd 2D Lookup Table/1
  PIDF Controller Va_theta Ki 2D Lookup Table/1 -> PIDF Controller Va_theta/3(I), PIDF Controller Va_theta Kt Tracking Gain Scalar/1
  PIDF Controller Va_theta Kd 2D Lookup Table/1 -> PIDF Controller Va_theta/4(D)
  PIDF Controller Va_theta N 2D Lookup Table/1 -> PIDF Controller Va_theta/5(N)
  alpha/1 -> PIDF Controller Va_theta Kp 2D Lookup Table/2, PIDF Controller Va_theta Ki 2D Lookup Table/2, PIDF Controller Va_theta N 2D Lookup Table/2, PIDF Controller Va_theta Kd 2D Lookup Table/2
  Sign Inversion/1 -> Zero-Order Hold/1
  TR/1 -> Tracking Sign Inversion/1
  PIDF Controller Va_theta Kt Tracking Gain Scalar/1 -> PIDF Controller Va_theta/6(Kt)
  Tracking Sign Inversion/1 -> PIDF Controller Va_theta/7(TR)
  Zero-Order Hold/1 -> theta_c_Va/1

== system SkywalkerX8_Control_Digital/Autopilot/Gain Scheduled Controller h_theta Digital ==
  note: We know that wings-level trim has the aircraft with a pitch angle. As such,
      | we know that at a minimum this controller has to be a PI controller, because otherwise
      | we have no state to hold the required steady state theta command.
  h_e : Inport
  TR : Inport  Port=2
  Kd : Constant  Value=SkywalkerX8.Control.Longitudinal.altController.Digital.KdAlt(5, 3)
  Ki : Constant  Value=SkywalkerX8.Control.Longitudinal.altController.Digital.KiAlt(5, 3)
  Kp : Constant  Value=SkywalkerX8.Control.Longitudinal.altController.Digital.KpAlt(5, 3)
  Kt : Constant  Value=SkywalkerX8.Control.Longitudinal.altController.KtScalar*SkywalkerX8.Control.Longitudinal.altController.Digital.KiAlt(5, 3)
  N : Constant  Value=SkywalkerX8.Control.Longitudinal.altController.Digital.NAlt(5, 3)
  PIDF Controller h_theta : Subsystem
  Zero-Order Hold : ZeroOrderHold  SampleTime=SkywalkerX8.Control.Longitudinal.altController.Digital.SampleTime
  theta_c_h : Outport
  wires:
  Kp/1 -> PIDF Controller h_theta/2(P)
  h_e/1 -> PIDF Controller h_theta/1(u)
  Kd/1 -> PIDF Controller h_theta/4(D)
  N/1 -> PIDF Controller h_theta/5(N)
  PIDF Controller h_theta/1(y) -> Zero-Order Hold/1
  TR/1 -> PIDF Controller h_theta/7(TR)
  Ki/1 -> PIDF Controller h_theta/3(I)
  Kt/1 -> PIDF Controller h_theta/6(Kt)
  Zero-Order Hold/1 -> theta_c_h/1

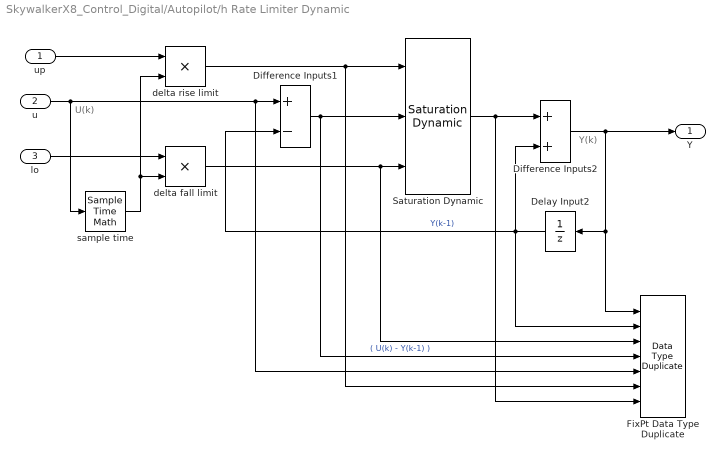
== system SkywalkerX8_Control_Digital/Autopilot/h Rate Limiter Dynamic ==
  note: U(k)
  note: Y(k)
  up : Inport
  u : Inport  Port=2
  lo : Inport  Port=3
  Delay Input2 : UnitDelay  Description=Store in Global RAM  DisableCoverage=on  InitialCondition=initOutput  SampleTime=-1
  Difference Inputs1 : Sum  Description=Add in CPU  DisableCoverage=on  Inputs=+-  OutDataTypeStr=Inherit: Inherit via back propagation
  Difference Inputs2 : Sum  Description=Add in CPU  OutDataTypeStr=Inherit: Inherit via back propagation
  FixPt Data Type Duplicate : DataTypeDuplicate  DisableCoverage=on  NumInputPorts=7
  Saturation Dynamic : simulink/Discontinuities/Saturation Dynamic  OutMin=[]  OutMax=[]  OutDataTypeStr=Inherit: Same as second input  OutDataType=fixdt(1, 16)  OutScaling=2^-10  DoSatur=off
  delta fall limit : Product  DisableCoverage=on  Inputs=**  OutDataTypeStr=Inherit: Inherit via back propagation  SaturateOnIntegerOverflow=on
  delta rise limit : Product  DisableCoverage=on  Inputs=**  OutDataTypeStr=Inherit: Inherit via back propagation  SaturateOnIntegerOverflow=on
  sample time : SampleTimeMath  DisableCoverage=on  TsampMathOp=Ts Only  weightValue=1
  Y : Outport  InitialOutput=0
  wires:
  Delay Input2/1 -> Difference Inputs1/2, FixPt Data Type Duplicate/2, Difference Inputs2/2  "Y(k-1)"
  Difference Inputs1/1 -> FixPt Data Type Duplicate/4, Saturation Dynamic/2  "( U(k) - Y(k-1) )"
  Difference Inputs2/1 -> Y/1, Delay Input2/1, FixPt Data Type Duplicate/1
  u/1 -> Difference Inputs1/1, FixPt Data Type Duplicate/5, sample time/1
  delta fall limit/1 -> FixPt Data Type Duplicate/3, Saturation Dynamic/3
  sample time/1 -> delta fall limit/2, delta rise limit/2
  Saturation Dynamic/1 -> Difference Inputs2/1, FixPt Data Type Duplicate/7
  delta rise limit/1 -> FixPt Data Type Duplicate/6, Saturation Dynamic/1
  lo/1 -> delta fall limit/1
  up/1 -> delta rise limit/1

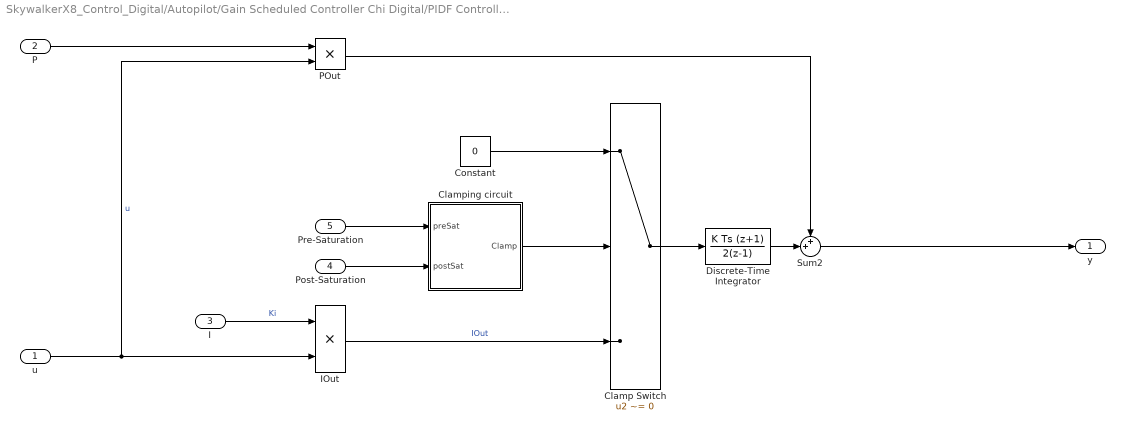
== system SkywalkerX8_Control_Digital/Autopilot/Gain Scheduled Controller Chi Digital/PIDF Controller Va_theta ==
  u : Inport
  P : Inport  Port=2
  I : Inport  Port=3
  Post-Saturation : Inport  Port=4
  Pre-Saturation : Inport  Port=5
  Clamp Switch : Switch  Criteria=u2 ~= 0
  Clamping circuit : Subsystem
  Constant : Constant  Value=0
  Discrete-Time Integrator : DiscreteIntegrator  IntegratorMethod=Integration: Trapezoidal  InitialCondition=SkywalkerX8.InitialConditions.PhiThetaPsi(1)  SampleTime=SkywalkerX8.Control.Lateral.ChiController.Digital.SampleTime  ICPrevOutput=DiscIntNeverNeededParam  ICPrevScaledInput=DiscIntNeverNeededParam
  IOut : Product  DisableCoverage=on
  POut : Product
  Sum2 : Sum  Inputs=++|
  y : Outport  InitialOutput=0
  wires:
  Sum2/1 -> y/1
  POut/1 -> Sum2/1
  u/1 -> POut/2, IOut/2  "u"
  Clamp Switch/1 -> Discrete-Time Integrator/1
  Discrete-Time Integrator/1 -> Sum2/2
  Constant/1 -> Clamp Switch/1
  I/1 -> IOut/1  "Ki"
  IOut/1 -> Clamp Switch/3  "IOut"
  Clamping circuit/1(Clamp) -> Clamp Switch/2
  P/1 -> POut/1
  Pre-Saturation/1 -> Clamping circuit/1(preSat)
  Post-Saturation/1 -> Clamping circuit/2(postSat)

== system SkywalkerX8_Control_Digital/Autopilot/Gain Scheduled Controller Phi Digital/DF Controller Phi ==
  N : Inport
  D : Inport  Port=2
  du/dt : Inport  Port=3
  Discrete-Time Integrator : DiscreteIntegrator  IntegratorMethod=Integration: Trapezoidal  SampleTime=SkywalkerX8.Control.Lateral.PhiController.Digital.SampleTime  ICPrevOutput=DiscIntNeverNeededParam  ICPrevScaledInput=DiscIntNeverNeededParam
  Product : Product
  Product1 : Product
  Sum : Sum  Inputs=|+-
  da* : Outport
  wires:
  Discrete-Time Integrator/1 -> da*/1, Sum/2  "da*"
  Product1/1 -> Discrete-Time Integrator/1  "Nda*_e"
  du/dt/1 -> Product/2
  D/1 -> Product/1
  Sum/1 -> Product1/2  "da*_e"
  N/1 -> Product1/1
  Product/1 -> Sum/1

== system SkywalkerX8_Control_Digital/Autopilot/Gain Scheduled Controller Phi Digital/PDF Controller Phi 2DOF ==
  u : Inport
  P : Inport  Port=2
  D : Inport  Port=3
  N : Inport  Port=4
  Discrete-Time Integrator : DiscreteIntegrator  SampleTime=SkywalkerX8.Control.Lateral.PhiController.Digital.SampleTime  ICPrevOutput=DiscIntNeverNeededParam  ICPrevScaledInput=DiscIntNeverNeededParam
  POut : Product
  Product : Product
  Product1 : Product
  Sum : Sum  Inputs=|+-
  Sum2 : Sum
  y : Outport  InitialOutput=0
  wires:
  Sum2/1 -> y/1
  N/1 -> Product1/1
  Product1/1 -> Discrete-Time Integrator/1, Sum2/2
  Sum/1 -> Product1/2
  POut/1 -> Sum2/1
  D/1 -> Product/2
  u/1 -> Product/1, POut/2  "u"
  Discrete-Time Integrator/1 -> Sum/2
  Product/1 -> Sum/1
  P/1 -> POut/1

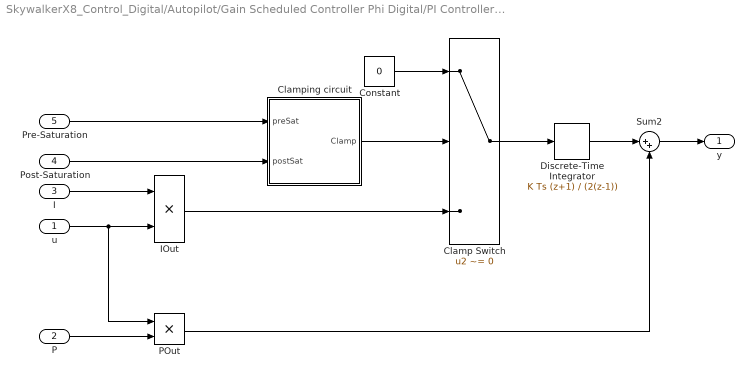
== system SkywalkerX8_Control_Digital/Autopilot/Gain Scheduled Controller Phi Digital/PI Controller Phi ==
  u : Inport
  P : Inport  Port=2
  I : Inport  Port=3
  Post-Saturation : Inport  Port=4
  Pre-Saturation : Inport  Port=5
  Clamp Switch : Switch  Criteria=u2 ~= 0
  Clamping circuit : Subsystem
  Constant : Constant  Value=0
  Discrete-Time Integrator : DiscreteIntegrator  IntegratorMethod=Integration: Trapezoidal  InitialCondition=SkywalkerX8.InitialConditions.da  SampleTime=SkywalkerX8.Control.Lateral.PhiController.Digital.SampleTime  ICPrevOutput=DiscIntNeverNeededParam  ICPrevScaledInput=DiscIntNeverNeededParam
  IOut : Product  DisableCoverage=on
  POut : Product
  Sum2 : Sum  Inputs=|++
  y : Outport  InitialOutput=0
  wires:
  IOut/1 -> Clamp Switch/3
  Clamp Switch/1 -> Discrete-Time Integrator/1
  Sum2/1 -> y/1
  Pre-Saturation/1 -> Clamping circuit/1(preSat)
  Post-Saturation/1 -> Clamping circuit/2(postSat)
  Clamping circuit/1(Clamp) -> Clamp Switch/2
  Constant/1 -> Clamp Switch/1
  Discrete-Time Integrator/1 -> Sum2/1
  POut/1 -> Sum2/2
  P/1 -> POut/2
  u/1 -> POut/1, IOut/2
  I/1 -> IOut/1

== system SkywalkerX8_Control_Digital/Autopilot/Gain Scheduled Controller Theta Digital/DF Controller Theta ==
  N : Inport
  D : Inport  Port=2
  du/dt : Inport  Port=3
  Discrete-Time Integrator : DiscreteIntegrator  IntegratorMethod=Integration: Trapezoidal  SampleTime=SkywalkerX8.Control.Longitudinal.thetaController.Digital.SampleTime  ICPrevOutput=DiscIntNeverNeededParam  ICPrevScaledInput=DiscIntNeverNeededParam
  Product : Product
  Product1 : Product
  Sum : Sum  Inputs=|+-
  de* : Outport
  wires:
  Discrete-Time Integrator/1 -> de*/1, Sum/2  "de*"
  Product1/1 -> Discrete-Time Integrator/1  "Nde*_e"
  du/dt/1 -> Product/2
  D/1 -> Product/1
  Sum/1 -> Product1/2  "de*_e"
  N/1 -> Product1/1
  Product/1 -> Sum/1
